simulink model "ctrlSys_vi"  (R2025b)
settings: Solver=ode14x  StartTime=0.0  StopTime=400  FixedStep=Ts_local  RelTol=1e-4
model workspace (MAT data in the model file):
  CtrlChoice = "MPC_QP"
values from neighbouring files (symbols this model uses):
  Ts_ctrl = 0.1    [ctrlSys.sldd]
undefined symbols (not defined in the file or in its folder): v_lb, v_ub
libraries: simulink x3, slpidlib x1
settings Model: DataDictionary=ctrlSys.sldd  SimulationMode=accelerator  Creator=LYG  LastModifiedBy=i336
settings SolverCC: ZeroCrossControl=DisableAll

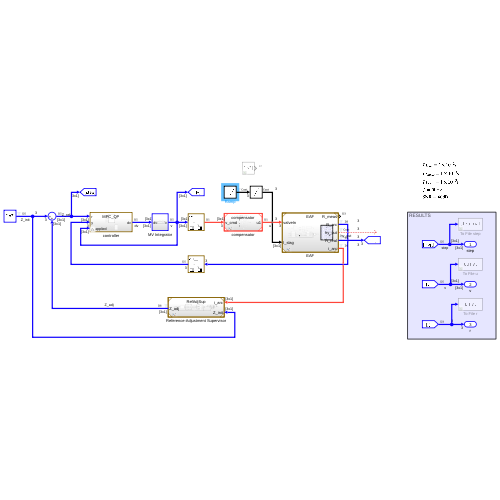
[thumbnail: Simulink's stored preview of the top-level diagram]
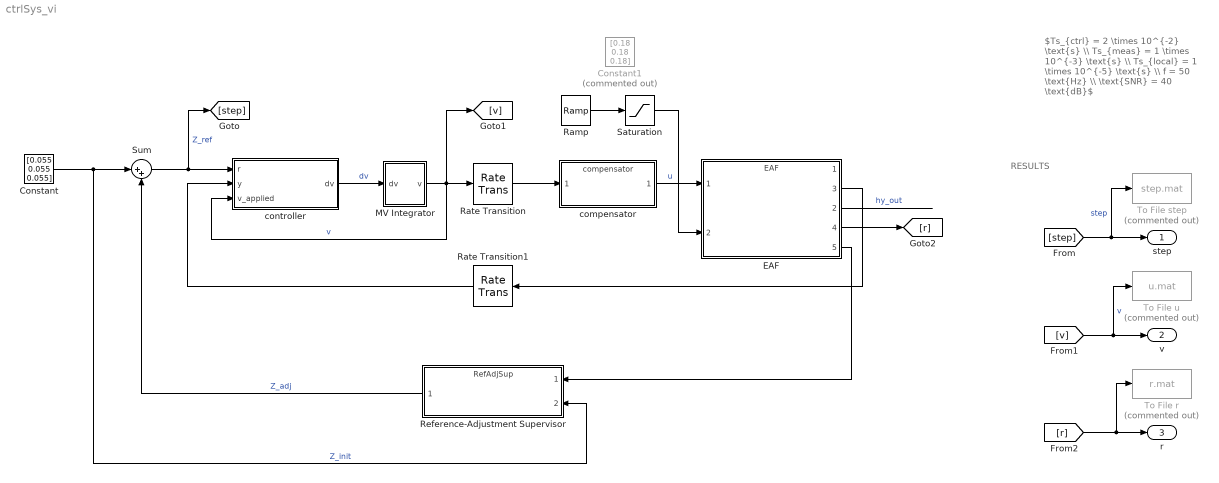
== system ctrlSys_vi ==
  note: RESULTS
  note: $Ts_{ctrl} = 2 \times 10^{-2} \text{s} \\ Ts_{meas} = 1 \times 10^{-3} \text{s} \\ Ts_{local} = 1 \times 10^{-5} \text{s} \\ f = 50 \text{Hz} \\ \text{SNR} = 40 \text{dB}$
  Constant : Constant  Value=[0.055 0.055 0.055]  SampleTime=Ts_ctrl
  Constant1 : Constant  Commented=on  Value=[0.18 0.18 0.18]
  EAF : ModelReference  ModelNameDialog=EAF.slx  SimulationMode=Normal  ModelReferenceVersion=1.100
      settings: PortSchema="{\"entries\":[{\"content\":{\"sides\":[{\"content\":{\"connectorIds\":[\"In1\",\"In2\"]},\"type\":\"ConnectorPlacement.EquallySpacedRectSide\",\"uuid\":\"d86d1ee9-bc46-42a8-9524-fd49ad5347e3\"},{\"content\":{\"connectorIds\":[\"Out1\",\"Out3\",\"Out2\",\"Out4\",\"Out5\"],\"side\":\"RIGHT\"},\"type\":\"ConnectorPlacement.EquallySpacedRectSide\",\"uuid\":\"5e39bbbf-7cf1-43cf-875a-d495ff7677ac\"},{\"content\":{\"side\":\"TOP\"},\"type\":\"ConnectorPlacement.EquallySpacedRectSide\",\"uuid\":\"55c1c4d1-73d3-4709-8e13-d53b4be02911\"}]},\"type\":\"ConnectorPlacement.EquallySpacedConnector\",\"uuid\":\"f9fda77e-4610-4959-9334-0640198713a5\"}],\"packageUris\":[\"http://schema.mathworks.com/mf0/Connector/R2020b\"],\"version\":\"1.0\"}"
  MV Integrator : Subsystem
  Ramp : simulink/Sources/Ramp  slope=(0.21 - 0.18) / (350 - 50)  start=[50 50 50]  InitialOutput=0.18
  Rate Transition : RateTransition  OutPortSampleTime=Ts_local
  Rate Transition1 : RateTransition  OutPortSampleTime=Ts_ctrl
  Reference-Adjustment Supervisor : ModelReference  ModelNameDialog=RefAdjSup.slx  SimulationMode=Normal  ModelReferenceVersion=1.57
  Saturation : Saturate  UpperLimit=0.21  LowerLimit=0
  Sum : Sum  Inputs=|++
  To File r : ToFile  Commented=on  Filename=r.mat  MatrixName=r  SaveFormat=Timeseries
  To File step : ToFile  Commented=on  Filename=step.mat  MatrixName=step  SaveFormat=Timeseries
  To File u : ToFile  Commented=on  Filename=u.mat  MatrixName=u  SaveFormat=Timeseries
  compensator : ModelReference  ModelNameDialog=compensator.slx  SimulationMode=Normal  ModelReferenceVersion=1.24
  controller : Subsystem  Variant=on
  step : Outport
  v : Outport  Port=2
  r : Outport  Port=3
  wires:
  [step] -> To File step/1, step/1  "step"
  [v] -> To File u/1, v/1  "v"
  [r] -> To File r/1, r/1
  Rate Transition/1 -> compensator/1
  compensator/1 -> EAF/1  "u"
  EAF/3 -> Rate Transition1/1
  EAF/4 -> [r]
  Rate Transition1/1 -> controller/2(y)
  MV Integrator/1(v) -> [v], controller/3(v_applied), Rate Transition/1  "v"
  controller/1(dv) -> MV Integrator/1(dv)  "dv"
  Sum/1 -> [step], controller/1(r)  "Z_ref"
  Constant/1 -> Reference-Adjustment Supervisor/2, Sum/1  "Z_init"
  Reference-Adjustment Supervisor/1 -> Sum/2  "Z_adj"
  EAF/5 -> Reference-Adjustment Supervisor/1
  EAF/2 -> ?  "hy_out"
  Ramp/1 -> Saturation/1
  Saturation/1 -> EAF/2

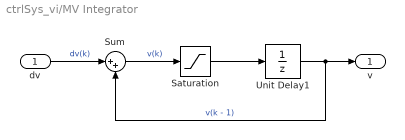
== system ctrlSys_vi/MV Integrator ==
  dv : Inport
  Saturation : Saturate  UpperLimit=v_ub  LowerLimit=v_lb
  Sum : Sum  Inputs=|++
  Unit Delay1 : UnitDelay  SampleTime=-1  HasFrameUpgradeWarning=on
  v : Outport
  wires:
  Saturation/1 -> Unit Delay1/1
  Unit Delay1/1 -> v/1, Sum/2  "v(k - 1)"
  dv/1 -> Sum/1  "dv(k)"
  Sum/1 -> Saturation/1  "v(k)"

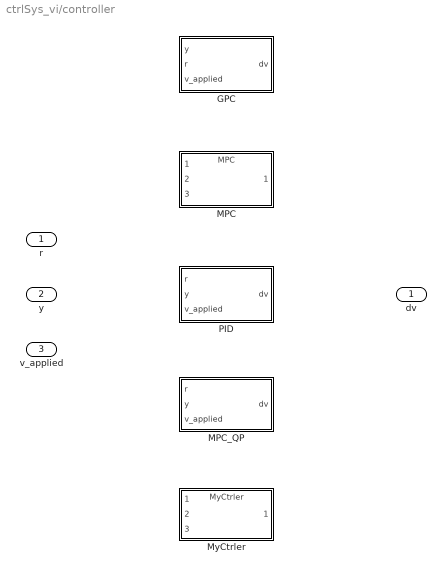
== system ctrlSys_vi/controller ==
  r : Inport
  y : Inport  Port=2
  v_applied : Inport  Port=3
  GPC : Subsystem  VariantControl="CtrlChoice == \"GPC\""
  MPC : ModelReference  ModelNameDialog=MPC.slx  VariantControl="CtrlChoice == \"MPC\""  ModelReferenceVersion=1.9
  MPC_QP : Subsystem  VariantControl="CtrlChoice == \"MPC_QP\""
  MyCtrler : ModelReference  ModelNameDialog=MyCtrler.slx  SimulationMode=Normal  VariantControl="CtrlChoice == \"MyCtrler\""  ModelReferenceVersion=1.44
  PID : Subsystem  VariantControl="CtrlChoice == \"PID\""
  dv : Outport

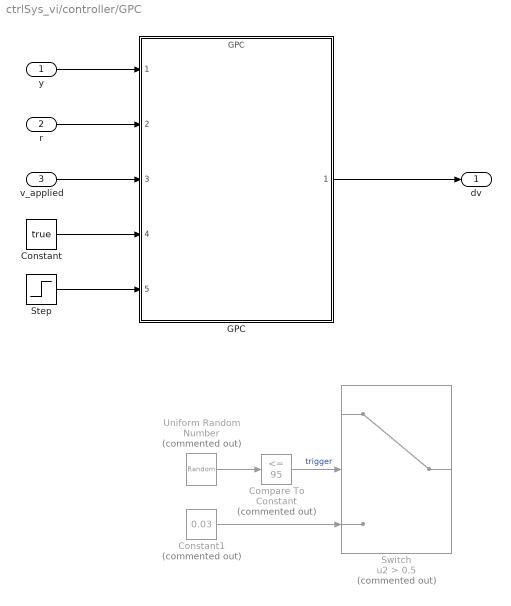
== system ctrlSys_vi/controller/GPC ==
  y : Inport
  r : Inport  Port=2
  v_applied : Inport  Port=3
  Compare To Constant : simulink/Logic and Bit Operations/Compare To Constant  Commented=on  relop=<=  const=95  OutDataTypeStr=boolean
  Constant : Constant  Value=true
  Constant1 : Constant  Commented=on  Value=0.03  SampleTime=Ts_ctrl
  GPC : ModelReference  ModelNameDialog=GPC.slx  SimulationMode=Normal  ModelReferenceVersion=1.264
  Step : Step  Time=0.1  Before=1  After=0  SampleTime=Ts_ctrl
  Switch : Switch  Commented=on  Criteria=u2 > Threshold  Threshold=0.5  SaturateOnIntegerOverflow=off  InputSameDT=off
  Uniform Random Number : UniformRandomNumber  Commented=on  Minimum=0  Maximum=100  SampleTime=Ts_ctrl * 5
  dv : Outport
  wires:
  v_applied/1 -> GPC/3
  r/1 -> GPC/2
  y/1 -> GPC/1
  Step/1 -> GPC/5
  GPC/1 -> dv/1
  Constant/1 -> GPC/4
  Compare To Constant/1 -> Switch/2  "trigger"
  Uniform Random Number/1 -> Compare To Constant/1
  Constant1/1 -> Switch/3

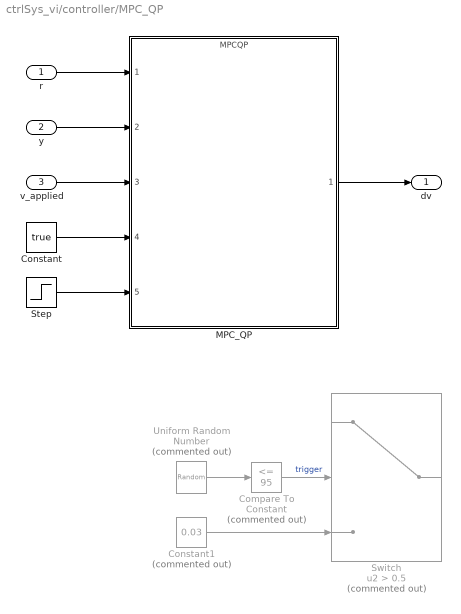
== system ctrlSys_vi/controller/MPC_QP ==
  r : Inport
  y : Inport  Port=2
  v_applied : Inport  Port=3
  Compare To Constant : simulink/Logic and Bit Operations/Compare To Constant  Commented=on  relop=<=  const=95  OutDataTypeStr=boolean
  Constant : Constant  Value=true
  Constant1 : Constant  Commented=on  Value=0.03  SampleTime=Ts_ctrl
  MPC_QP : ModelReference  ModelNameDialog=MPCQP.slx  SimulationMode=Normal  ModelReferenceVersion=1.59
  Step : Step  Time=0.1  Before=1  After=0  SampleTime=Ts_ctrl
  Switch : Switch  Commented=on  Criteria=u2 > Threshold  Threshold=0.5  SaturateOnIntegerOverflow=off  InputSameDT=off
  Uniform Random Number : UniformRandomNumber  Commented=on  Minimum=0  Maximum=100  SampleTime=Ts_ctrl * 5
  dv : Outport
  wires:
  r/1 -> MPC_QP/1
  v_applied/1 -> MPC_QP/3
  y/1 -> MPC_QP/2
  MPC_QP/1 -> dv/1
  Compare To Constant/1 -> Switch/2  "trigger"
  Uniform Random Number/1 -> Compare To Constant/1
  Constant1/1 -> Switch/3
  Constant/1 -> MPC_QP/4
  Step/1 -> MPC_QP/5

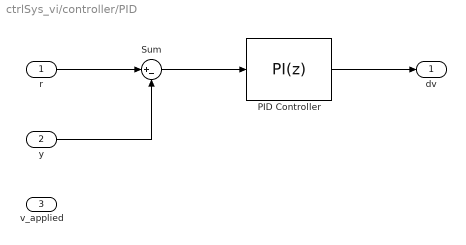
== system ctrlSys_vi/controller/PID ==
  r : Inport
  y : Inport  Port=2
  v_applied : Inport  Port=3
  PID Controller : slpidlib/PID Controller  Controller=PI  Form=Parallel  TimeDomain=Discrete-time  UseExternalTs=off  SampleTime=Ts_ctrl  IntegratorMethod=Forward Euler  FilterMethod=Forward Euler  ControllerParametersSource=internal  P=100  I=10  UseKiTs=off  D=0  UseExternalDerivativeSource=off  N=100  UseFilter=on  TunerSelectOption=Transfer Function Based (PID Tuner App)  InitialConditionSource=internal  InitialConditionForIntegrator=0  InitialConditionForFilter=0  DifferentiatorICPrevScaledInput=0  ExternalReset=none  TrackingMode=off  Kt=1  LimitOutput=off  SatLimitsSource=internal  UpperSaturationLimit=inf  LowerSaturationLimit=-inf  LinearizeAsGain=on  AntiWindupMode=none  Kb=1  LimitIntegrator=off  UpperIntegratorSaturationLimit=inf  LowerIntegratorSaturationLimit=-inf  POutMin=[]  POutMax=[]  IOutMin=[]  IOutMax=[]  DOutMin=[]  DOutMax=[]  NOutMin=[]  NOutMax=[]  SumOutMin=[]  SumOutMax=[]  SaturationOutMin=[]  SaturationOutMax=[]  PParamMin=[]  PParamMax=[]  IParamMin=[]  IParamMax=[]  DParamMin=[]  DParamMax=[]  NParamMin=[]  NParamMax=[]  KbParamMin=[]  KbParamMax=[]  KtParamMin=[]  KtParamMax=[]  KbOutMin=[]  KbOutMax=[]  KtOutMin=[]  KtOutMax=[]  IntegratorOutMin=[]  IntegratorOutMax=[]  FilterOutMin=[]  FilterOutMax=[]  SumI1OutMin=[]  SumI1OutMax=[]  SumI2OutMin=[]  SumI2OutMax=[]  SumI3OutMin=[]  SumI3OutMax=[]  SumI4OutMin=[]  SumI4OutMax=[]  SumDOutMin=[]  SumDOutMax=[]  DifferentiatorOutMin=[]  DifferentiatorOutMax=[]  FilterDiffOutCoefMin=[]  FilterDiffOutCoefMax=[]  ReciprocalOutMin=[]  ReciprocalOutMax=[]  SumDenOutMin=[]  SumDenOutMax=[]  SumNumOutMin=[]  SumNumOutMax=[]  DivideOutMin=[]  DivideOutMax=[]  UdiffTsProdOutMin=[]  UdiffTsProdOutMax=[]  NTsProdOutMin=[]  NTsProdOutMax=[]  UintegralTsProdOutMin=[]  UintegralTsProdOutMax=[]  UngainTsProdOutMin=[]  UngainTsProdOutMax=[]  ClampingZeroOutDataTypeStr=Inherit: Inherit via back propagation  ClampingZeroOutMin=[]  ClampingZeroOutMax=[]  FilterDenConstantOutDataTypeStr=Inherit: Inherit via back propagation  FilterDenConstantOutMin=[]  FilterDenConstantOutMax=[]  PCopyOutDataTypeStr=Inherit: Inherit via back propagation  PCopyOutMin=[]  PCopyOutMax=[]  NCopyOutDataTypeStr=Inherit: Inherit via back propagation  NCopyOutMin=[]  NCopyOutMax=[]  IntegratorContinuousStateAttributes=''  IntegratorStateMustResolveToSignalObject=off  IntegratorRTWStateStorageClass=Auto  FilterContinuousStateAttributes=''  FilterStateMustResolveToSignalObject=off  FilterRTWStateStorageClass=Auto  ParallelPVariant=InternalParameters  IdealPVariant=Disabled  IVariant=InternalParameters  DVariant=Disabled  IntegratorVariant=Discrete  SatVariant=Disabled  AWVariant=Passthrough  PCopyVariant=Disabled  TRVariant=Disabled  FdbkBlocksVariant=Forward  IdealPFdbkVariant=Disabled  SatFdbkVariant=Disabled  DerivativeFilterVariant=Disabled  NVariant=Disabled  NCopyVariant=Disabled_SignalSpec  FilterICVariant=Disabled  IntegratorICVariant=InternalICs  ExternalResetVariant=Disabled  TRSumVariant=Passthrough  SumFdbkVariant=Disabled  SumVariant=Sum_PI  TsampFilterVariant=InternalTs  TsampNgainVariant=Passthrough  TsampIntegralVariant=Disabled_SignalSpec  ExternalSaturationOutDataTypeStr=Inherit: Same as second input  DerivativeSourceVariant=Disabled  PreIntVariant=InternalPreInt
  Sum : Sum  Inputs=|+-
  dv : Outport
  wires:
  r/1 -> Sum/1
  Sum/1 -> PID Controller/1
  y/1 -> Sum/2
  PID Controller/1 -> dv/1
